simulink subsystem "subsPreprocesado"  (R2021b)
settings: Solver=VariableStepAuto  StartTime=0.0  StopTime=10.0  RelTol=1e-3
undefined symbols (not defined in the file): fdesignblkfcn, gcbh
libraries: dsparch4 x2
settings Model: Creator=alvaro  LastModifiedBy=alvaro

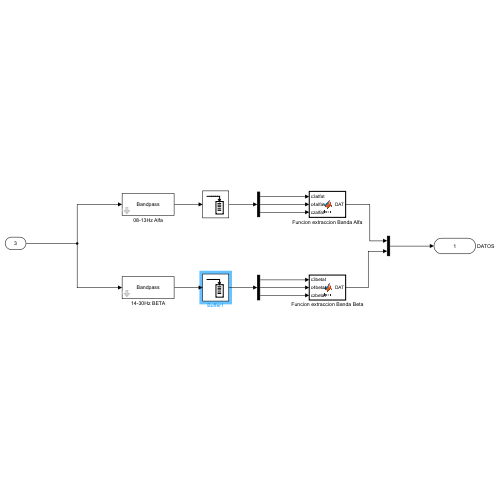
[thumbnail: Simulink's stored preview of the top-level diagram]
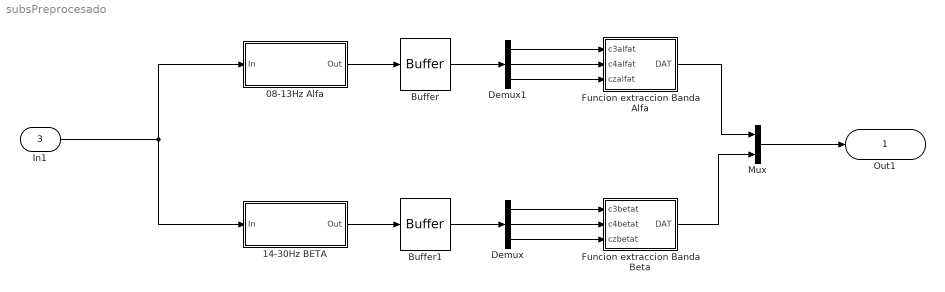
== system subsPreprocesado ==
  In1 : Inport  Port=3
  08-13Hz Alfa : Subsystem  DialogController=fdesignblkfcn  InitFcn=fdesignblkfcn(gcbh, {'InitFcn'});  mask(Bandpass Filter){}
      mask help: Design a bandpass filter
      settings: CopyFcn=fdesignblkfcn(gcbh, {'CopyFcn'});
      mask Help: helpview(mapfilelocation('dsp'), 'dspbandpassfilter');
      mask Display: disp('Bandpass');
  14-30Hz BETA : Subsystem  DialogController=fdesignblkfcn  InitFcn=fdesignblkfcn(gcbh, {'InitFcn'});  mask(Bandpass Filter){}
      mask help: Design a bandpass filter
      settings: CopyFcn=fdesignblkfcn(gcbh, {'CopyFcn'});
      mask Help: helpview(mapfilelocation('dsp'), 'dspbandpassfilter');
      mask Display: disp('Bandpass');
  Buffer : Buffer  N=250  OutputFrames=off
  Buffer1 : Buffer  N=250  OutputFrames=off
  Demux : Demux  Outputs=3
  Demux1 : Demux  Outputs=3
  Funcion extraccion Banda Alfa : MATLAB Function  TreatAsAtomicUnit=on
  Funcion extraccion Banda Beta : MATLAB Function  TreatAsAtomicUnit=on
  Mux : Mux  Inputs=2
  Out1 : Outport  SignalName=DATOS
  wires:
  Funcion extraccion Banda Beta/1(DAT) -> Mux/2
  Funcion extraccion Banda Alfa/1(DAT) -> Mux/1
  Demux/2 -> Funcion extraccion Banda Beta/2(c4betat)
  Demux/1 -> Funcion extraccion Banda Beta/1(c3betat)
  14-30Hz BETA/1(Out) -> Buffer1/1
  08-13Hz Alfa/1(Out) -> Buffer/1
  Demux/3 -> Funcion extraccion Banda Beta/3(czbetat)
  Demux1/2 -> Funcion extraccion Banda Alfa/2(c4alfat)
  Demux1/1 -> Funcion extraccion Banda Alfa/1(c3alfat)
  Demux1/3 -> Funcion extraccion Banda Alfa/3(czalfat)
  In1/1 -> 14-30Hz BETA/1(In), 08-13Hz Alfa/1(In)
  Mux/1 -> Out1/1
  Buffer/1 -> Demux1/1
  Buffer1/1 -> Demux/1

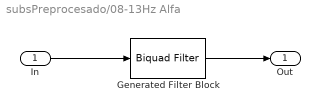
== system subsPreprocesado/08-13Hz Alfa ==
  In : Inport
  Generated Filter Block : dsparch4/Biquad Filter  Tag=BlockMethodSubSystem  FilterSource=Dialog parameters  CoeffSource=Specify via dialog  FilterObject=BQF  IIRFiltStruct=Direct form II  BiQuadCoeffs=[0.0704460167105730589 0 -0.0704460167105730589 1 -1.83801933650841587 0.892367175066100304;0.0183579484604002446 0 -0.0183579484604002446 1 -1.80862098101568658 0.878586422262470301;0.149249557305678987 0 -0.149249557305678987 1 -1.93478463247681454 0.975190357482606518;0.036212676387558311 0 -0.036212676387558311 1 -1.858817963856779 0.961003298692826524;0.120268292464888585 0 -0.120268292464888585 1 -1.88439409475496844 0.928883949733004255;2 0 -2 1 -1.81326187630040003 0.901276904931625489]  ScaleValues=[0.0249077373068375546;1;1;1;1;1;1.16150950971942923]  IC=0  ICnum=0  ICden=0  a0Flag=Warning  optimizeScaleValues=on  ScaleValueMode=Specify via input port (g)  roundingMode=Floor  overflowMode=off  scaleValueFracLength=14  denProdOutputFracLength=30  denAccumFracLength=30  secondMemoryFracLength=15
  Out : Outport
  wires:
  In/1 -> Generated Filter Block/1
  Generated Filter Block/1 -> Out/1

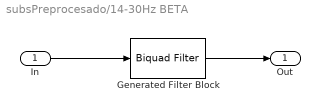
== system subsPreprocesado/14-30Hz BETA ==
  In : Inport
  Generated Filter Block : dsparch4/Biquad Filter  Tag=BlockMethodSubSystem  FilterSource=Dialog parameters  CoeffSource=Specify via dialog  FilterObject=BQF  IIRFiltStruct=Direct form II  BiQuadCoeffs=[0.0704460167105730589 0 -0.0704460167105730589 1 -1.83801933650841587 0.892367175066100304;0.0183579484604002446 0 -0.0183579484604002446 1 -1.80862098101568658 0.878586422262470301;0.149249557305678987 0 -0.149249557305678987 1 -1.93478463247681454 0.975190357482606518;0.036212676387558311 0 -0.036212676387558311 1 -1.858817963856779 0.961003298692826524;0.120268292464888585 0 -0.120268292464888585 1 -1.88439409475496844 0.928883949733004255;2 0 -2 1 -1.81326187630040003 0.901276904931625489]  ScaleValues=[0.0249077373068375546;1;1;1;1;1;1.16150950971942923]  IC=0  ICnum=0  ICden=0  a0Flag=Warning  optimizeScaleValues=on  ScaleValueMode=Specify via input port (g)  roundingMode=Floor  overflowMode=off  scaleValueFracLength=14  denProdOutputFracLength=30  denAccumFracLength=30  secondMemoryFracLength=15
  Out : Outport
  wires:
  In/1 -> Generated Filter Block/1
  Generated Filter Block/1 -> Out/1

== matlab function subsPreprocesado/Funcion extraccion Banda Alfa ==
  settings: updateMethod=DISCRETE  sampleTime=250
  data: c3alfat input; DAT output; c4alfat input; czalfat input
function DAT = fcn(c3alfat, c4alfat, czalfat)

%Funcion Wavalet para descomponer la señas y tener reducir el nº de muestras
[cc3 ,lc3]= wavedec(c3alfat,2,'db2');
[ccz ,lcz]= wavedec(czalfat,2,'db2');
[cc4 ,lc4]= wavedec(c4alfat,2,'db2');
c3alfat = appcoef(cc3,lc3,'db2'); 
czalfat = appcoef(ccz,lcz,'db2'); 
c4alfat = appcoef(cc4,lc4,'db2'); 

%Calculamos la Densidad espectral de Potencia mediante el metodo Welch 
[C3welchalfa,f] = pwelch(c3alfat);
f=(f/(2*pi))*60;
[Czwelchalfa,f] = pwelch(czalfat);
f=(f/(2*pi))*60;
[C4welchalfa,f] = pwelch(c4alfat);
f=(f/(2*pi))*60;

%Calculamos la FFT de la señal.
C3alfat = abs(fft(c3alfat)); 
Czalfat = abs(fft(czalfat));
C4alfat = abs(fft(c4alfat)); 

%%Extracion de Caracteristicas 
% Alfa 
C3VARa=var(C3alfat);
CzVARa=var(Czalfat);
C4VARa=var(C4alfat);
C3COVARa=cov(C3alfat);
CzCOVARa=cov(Czalfat);
C4COVARa=cov(C4alfat);
C3MEANa=cov(C3alfat);
CzMEANa=cov(Czalfat);
C4MEANa=cov(C4alfat);
C3STDa=std(C3alfat);
CzSTDa=std(Czalfat);
C4STDa=std(C4alfat);
C3MAXPSDa=max(C3welchalfa);
CzMAXPSDa=max(Czwelchalfa);
C4MAXPSDa=max(C4welchalfa);
c3VARa=var(c3alfat);
czVARa=var(czalfat);
c4VARa=var(c4alfat);
c3COVARa=cov(c3alfat);
czCOVARa=cov(czalfat);
c4COVARa=cov(c4alfat);
c3MEANa=cov(c3alfat);
czMEANa=cov(czalfat);
c4MEANa=cov(c4alfat);
c3STDa=std(c3alfat);
czSTDa=std(czalfat);
c4STDa=std(c4alfat);
c3MAXa=max(c3alfat);
czMAXa=max(czalfat);
c4MAXa=max(c4alfat);
c3MINa=min(c3alfat);
czMINa=min(czalfat);
c4MINa=min(c4alfat);

%Vector de caracteristicas 
DAT = [ C3VARa,C3COVARa,C3MEANa,C3STDa,C3MAXPSDa,c3VARa,c3COVARa,c3MEANa,c3STDa,c3MAXa,c3MINa,CzVARa,CzCOVARa,CzMEANa,CzMAXPSDa,CzSTDa,czVARa,czCOVARa,czMEANa,czSTDa,czMAXa,czMINa,C4VARa,C4COVARa,C4MEANa,C4MAXPSDa,C4STDa,c4VARa,c4COVARa,c4MEANa,c4STDa,c4MAXa,c4MINa];

== matlab function subsPreprocesado/Funcion extraccion Banda Beta ==
  settings: updateMethod=DISCRETE  sampleTime=250
  data: c3betat input; DAT output; c4betat input; czbetat input
function DAT = fcn(c3betat,c4betat,czbetat)

%Funcion Wavalet para descomponer la señas y tener reducir el nº de muestras
[cc3 ,lc3]= wavedec(c3betat,1,'db2');
[ccz ,lcz]= wavedec(czbetat,1,'db2');
[cc4 ,lc4]= wavedec(c4betat,1,'db2');
c3betat = appcoef(cc3,lc3,'db2'); 
czbetat = appcoef(ccz,lcz,'db2'); 
c4betat = appcoef(cc4,lc4,'db2'); 

%Calculamos la Densidad espectral de Potencia mediante el metodo Welc
[C3welchbeta,f] = pwelch(c3betat);
f=(f/(2*pi))*60;
[Czwelchbeta,f] = pwelch(czbetat);
f=(f/(2*pi))*60;
[C4welchbeta,f] = pwelch(c4betat);
f=(f/(2*pi))*60;

%Calculamos la FFT de la señal.
C3betat = abs(fft(c3betat)); 
Czbetat = abs(fft(czbetat));
C4betat = abs(fft(c4betat)); 


%%Extracion de Caracteristicas
%Beta
C3VARb=var(C3betat);
CzVARb=var(Czbetat);
C4VARb=var(C4betat);
C3COVARb=cov(C3betat);
CzCOVARb=cov(Czbetat);
C4COVARb=cov(C4betat);
C3MEANb=cov(C3betat);
CzMEANb=cov(Czbetat);
C4MEANb=cov(C4betat);
C3STDb=std(C3betat);
CzSTDb=std(Czbetat);
C4STDb=std(C4betat);
C3MAXPSDb=max(C3welchbeta);
CzMAXPSDb=max(Czwelchbeta);
C4MAXPSDb=max(C4welchbeta);
c3VARb=var(c3betat);
czVARb=var(czbetat);
c4VARb=var(c4betat);
c3COVARb=cov(c3betat);
czCOVARb=cov(czbetat);
c4COVARb=cov(c4betat);
c3MEANb=cov(c3betat);
czMEANb=cov(czbetat);
c4MEANb=cov(c4betat);
c3STDb=std(c3betat);
czSTDb=std(czbetat);
c4STDb=std(c4betat);
c3MAXb=max(c3betat);
czMAXb=max(czbetat);
c4MAXb=max(c4betat);
c3MINb=min(c3betat);
czMINb=min(czbetat);
c4MINb=min(c4betat);

DAT = [C3VARb,C3COVARb,C3MEANb,C3MAXPSDb,C3STDb,c3VARb,c3COVARb,c3MEANb,c3STDb,c3MAXb,c3MINb,CzVARb,CzCOVARb,CzMEANb,CzMAXPSDb,CzSTDb,czVARb,czCOVARb,czMEANb,czSTDb,czMAXb,czMINb,C4VARb,C4COVARb,C4MEANb,C4MAXPSDb,C4STDb,c4VARb,c4COVARb,c4MEANb,c4STDb,c4MAXb,c4MINb];
